simulink model "Smart_Servo_Test"  (R2022b)
settings: Solver=FixedStepAuto  StartTime=0.0  StopTime=10  FixedStep=1e-3  RelTol=1e-3  EnableMultiTasking=on
undefined symbols (not defined in the file or in its folder): AS5600, INA219
libraries: arduinolib x16, simulink x5, hdlsllib x2, dspsigops x2, simulink_extras x1, spsTriangleGeneratorLib x1
settings Model: ExtModeTrigDuration=2  Creator=gotta  LastModifiedBy=gotta
settings SolverCC: AutoInsertRateTranBlk=on
settings DataIOCC: SaveFormat=Array  SaveOutput=off  DSMLogging=off  SaveTime=off  ReturnWorkspaceOutputs=off
settings OptimizationCC: EnhancedBackFolding=on  PassReuseOutputArgsAs=Individual arguments  ZeroExternalMemoryAtStartup=off  ZeroInternalMemoryAtStartup=off  MaxStackSize=64  OptimizeBlockOrder=speed  DifferentSizesBufferReuse=on  OptimizationCustomize=off  EfficientTunableParamExpr=on
settings DebuggingCC: ParameterTunabilityLossMsg=error
settings HardwareCC: ProdBitPerPointer=32  ProdBitPerSizeT=32  ProdBitPerPtrDiffT=32  ProdLargestAtomicInteger=Long  ProdLargestAtomicFloat=Double  ProdWordSize=32  ProdHWDeviceType=ARM Compatible->ARM Cortex
settings SFSimCC: MATLABDynamicMemAlloc=off
settings RTWCC: Description=Embedded Coder  SystemTargetFile=ert.tlc  HardwareBoard=ESP32-WROOM(Arduino Compatible)  TLCOptions="-aInlineSetEventsForThisBaseRateFcn=TLC_FALSE -aSuppressMultiTaskScheduler=TLC_FALSE  -aRateBasedStepFcn=0"  TemplateMakefile=ert_default_tmf  Toolchain=ESP32  BuildConfiguration=Faster Runs
settings CodeAppCC: ForceParamTrailComments=on  IgnoreCustomStorageClasses=off  OperatorAnnotations=on  SimulinkDataObjDesc=on  SFDataObjDesc=on  InsertBlockDesc=on
settings ERTTargetCC: TargetLangStandard=C99 (ISO)  SupportContinuousTime=on  SupportVariableSizeSignals=on  ExtModeTransport=3  ExtModeStaticAlloc=on  ExtModeAutomaticAllocSize=off  ExtModeStaticAllocSize=65536  ExtModeMexFile=ext_xcp  ExtModeIntrfLevel=Level2 - Open

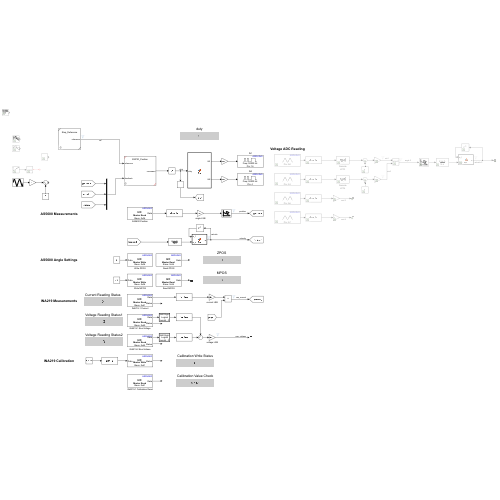
[thumbnail: Simulink's stored preview of the top-level diagram]
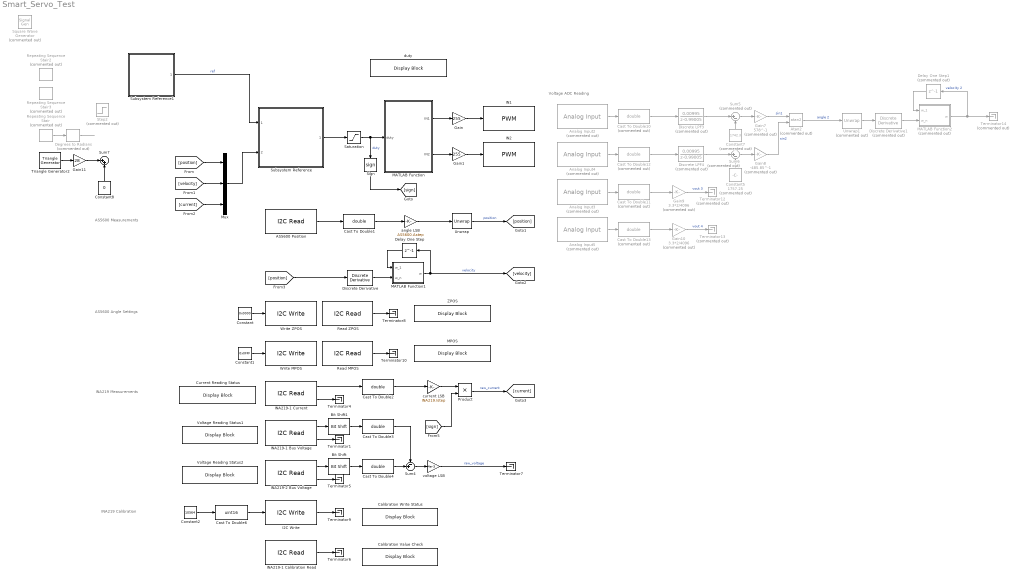
== system Smart_Servo_Test ==
  note: INA219 Calibration
  note: INA219 Measurements
  note: AS5600 Measurements
  note: Voltage ADC Reading
  note: AS5600 Angle Settings
  AS5600 Position : arduinolib/I2C Read  I2CModule=0  Mode=Master  SlaveAddress=AS5600.DEV_ADDR  SlaveByteOrder=BigEndian  Direction=Receiver  RegisterAddressMode=on  RegisterAddress=AS5600.ANGLE_ADDR  SlaveDataType=int16  DataLength=1  NoAck=off  RepeatedStart=off  OutputStatus=off  blockPlatform=ARDUINO  SampleTime=1e-3
  Analog Input2 : arduinolib/Analog Input  Commented=on  pinNumber=0  ReadResultsOnly=off  ConversionTriggerSource=Software  ExternalTriggerType=uint32( 0 )  OutputDataType=uint16  EnableConversionCompleteNotify=off  EnableOuputStatus=off  SampleTime=1e-3  blockPlatform=arduino
  Analog Input3 : arduinolib/Analog Input  Commented=on  pinNumber=6  ReadResultsOnly=off  ConversionTriggerSource=Software  ExternalTriggerType=uint32( 0 )  OutputDataType=uint16  EnableConversionCompleteNotify=off  EnableOuputStatus=off  SampleTime=1e-3  blockPlatform=arduino
  Analog Input4 : arduinolib/Analog Input  Commented=on  pinNumber=3  ReadResultsOnly=off  ConversionTriggerSource=Software  ExternalTriggerType=uint32( 0 )  OutputDataType=uint16  EnableConversionCompleteNotify=off  EnableOuputStatus=off  SampleTime=1e-3  blockPlatform=arduino
  Analog Input5 : arduinolib/Analog Input  Commented=on  pinNumber=7  ReadResultsOnly=off  ConversionTriggerSource=Software  ExternalTriggerType=uint32( 0 )  OutputDataType=uint16  EnableConversionCompleteNotify=off  EnableOuputStatus=off  SampleTime=1e-3  blockPlatform=arduino
  Atan2 : Trigonometry  Commented=on  Operator=atan2
  Bit Shift : hdlsllib/Logic and Bit Operations/Bit Shift  mode=Shift Right Logical  N=3
  Bit Shift1 : hdlsllib/Logic and Bit Operations/Bit Shift  mode=Shift Right Logical  N=3
  Calibration Value Check : DisplayBlock  LabelPosition=Hide  Transparency=1
  Calibration Write Status : DisplayBlock  LabelPosition=Hide  Transparency=1
  Cast To Double{1..4} (4 alike) : DataTypeConversion  OutDataTypeStr=double  SaturateOnIntegerOverflow=off  RndMeth=Floor
  Cast To Double{10..13} (4 alike) : DataTypeConversion  Commented=on  OutDataTypeStr=double  SaturateOnIntegerOverflow=off  RndMeth=Floor
  Cast To Double6 : DataTypeConversion  OutDataTypeStr=uint16  SaturateOnIntegerOverflow=off  RndMeth=Floor
  Constant : Constant  Value=0x0000
  Constant1 : Constant  Value=0x0FFF
  Constant2 : Constant  Value=10564  SampleTime=1e-3
  Constant5 : Constant  Commented=on  Value=1757.25
  Constant7 : Constant  Commented=on  Value=1742.3
  Constant8 : Constant  Value=0
  Current Reading Status : DisplayBlock  LabelPosition=Hide  Transparency=1
  Degrees to Radians : simulink_extras/Transformations/Degrees to Radians  Commented=on
  Delay One Step : Delay  DelayLength=1
  Delay One Step1 : Delay  Commented=on  DelayLength=1
  Discrete LPF3 : DiscreteTransferFcn  Commented=on  Numerator=[0.00995]  Denominator=[1 -0.99005]  SampleTime=1e-3
  Discrete LPF4 : DiscreteTransferFcn  Commented=on  Numerator=[0.00995]  Denominator=[1 -0.99005]  SampleTime=1e-3
  Discrete Derivative : simulink/Discrete/Discrete Derivative  gainval=1.0  ICPrevScaledInput=0.0  OutMin=[]  OutMax=[]  OutDataType=fixdt(1, 16)  OutScaling=2^-10  DoSatur=off
  Discrete Derivative1 : simulink/Discrete/Discrete Derivative  Commented=on  gainval=1.0  ICPrevScaledInput=0.0  OutMin=[]  OutMax=[]  OutDataType=fixdt(1, 16)  OutScaling=2^-10  DoSatur=off
  Gain : Gain  Gain=255
  Gain1 : Gain  Gain=255
  Gain10 : Gain  Commented=on  Gain=3.3*2/4096
  Gain11 : Gain  Gain=28
  Gain7 : Gain  Commented=on  Gain=578^-1
  Gain8 : Gain  Commented=on  Gain=-485.85^-1
  Gain9 : Gain  Commented=on  Gain=3.3*2/4096
  I2C Write : arduinolib/I2C Write  I2CModule=0  Mode=Master  SlaveAddress=0x41  SlaveByteOrder=BigEndian  Direction=Transmitter  RegisterAddressMode=on  RegisterAddress=INA219.CAL_ADDR  SlaveDataType=uint8  DataLength=1  NoAck=off  RepeatedStart=off  OutputStatus=on  blockPlatform=ARDUINO
  IN1 : arduinolib/PWM  pinNumber=16  frequencyType=Specify  desiredFrequency=5e4  achievableFrequency=50000
  IN2 : arduinolib/PWM  pinNumber=4  frequencyType=Specify  desiredFrequency=5e4  achievableFrequency=50000
  INA219-1 Bus Voltage : arduinolib/I2C Read  I2CModule=0  Mode=Master  SlaveAddress=0x40  SlaveByteOrder=BigEndian  Direction=Receiver  RegisterAddressMode=on  RegisterAddress=INA219.BV_ADDR  SlaveDataType=uint16  DataLength=1  NoAck=off  RepeatedStart=off  OutputStatus=on  blockPlatform=ARDUINO  SampleTime=1e-3
  INA219-1 Calibration Read : arduinolib/I2C Read  I2CModule=0  Mode=Master  SlaveAddress=0x41  SlaveByteOrder=BigEndian  Direction=Receiver  RegisterAddressMode=on  RegisterAddress=INA219.CAL_ADDR  SlaveDataType=int16  DataLength=1  NoAck=off  RepeatedStart=off  OutputStatus=off  blockPlatform=ARDUINO  SampleTime=1e-3
  INA219-1 Current : arduinolib/I2C Read  I2CModule=0  Mode=Master  SlaveAddress=0x41  SlaveByteOrder=BigEndian  Direction=Receiver  RegisterAddressMode=on  RegisterAddress=INA219.I_ADDR  SlaveDataType=int16  DataLength=1  NoAck=off  RepeatedStart=off  OutputStatus=on  blockPlatform=ARDUINO  SampleTime=1e-3
  INA219-2 Bus Voltage : arduinolib/I2C Read  I2CModule=0  Mode=Master  SlaveAddress=0x45  SlaveByteOrder=BigEndian  Direction=Receiver  RegisterAddressMode=on  RegisterAddress=INA219.BV_ADDR  SlaveDataType=uint16  DataLength=1  NoAck=off  RepeatedStart=off  OutputStatus=on  blockPlatform=ARDUINO  SampleTime=1e-3
  MATLAB Function : MATLAB Function  TreatAsAtomicUnit=on
  MATLAB Function1 : MATLAB Function  TreatAsAtomicUnit=on
  MATLAB Function2 : MATLAB Function  Commented=on  TreatAsAtomicUnit=on
  MPOS : DisplayBlock  LabelPosition=Hide  Transparency=1
  Mux : Mux  Inputs=3
  Product : Product
  Read MPOS : arduinolib/I2C Read  I2CModule=0  Mode=Master  SlaveAddress=AS5600.DEV_ADDR  SlaveByteOrder=BigEndian  Direction=Receiver  RegisterAddressMode=on  RegisterAddress=0X03  SlaveDataType=uint16  DataLength=1  NoAck=off  RepeatedStart=off  OutputStatus=off  blockPlatform=ARDUINO  SampleTime=1e-3
  Read ZPOS : arduinolib/I2C Read  I2CModule=0  Mode=Master  SlaveAddress=AS5600.DEV_ADDR  SlaveByteOrder=BigEndian  Direction=Receiver  RegisterAddressMode=on  RegisterAddress=0X01  SlaveDataType=uint16  DataLength=1  NoAck=off  RepeatedStart=off  OutputStatus=off  blockPlatform=ARDUINO  SampleTime=1e-3
  Repeating Sequence Stair : simulink/Sources/Repeating Sequence Stair  Commented=on  OutValues=2:2:360  tsamp=2  OutMin=[]  OutMax=[]  OutDataTypeStr=double  OutputDataTypeScalingMode=double  OutDataType=fixdt(0,8)  ConRadixGroup=Best Precision: Vector-wise  OutScaling=2^-12
  Repeating Sequence Stair2 : simulink/Sources/Repeating Sequence Stair  Commented=on  OutValues=[0.1:0.1:1, -[0.1:0.1:1]]  tsamp=10  OutMin=[]  OutMax=[]  OutDataTypeStr=double  OutputDataTypeScalingMode=double  OutDataType=fixdt(0,8)  ConRadixGroup=Best Precision: Vector-wise  OutScaling=2^-12
  Repeating Sequence Stair3 : simulink/Sources/Repeating Sequence Stair  Commented=on  OutValues=[0, 0.5:0.5:10, -[0.5:0.5:10]]  tsamp=5  OutMin=[]  OutMax=[]  OutDataTypeStr=double  OutputDataTypeScalingMode=double  OutDataType=fixdt(0,8)  ConRadixGroup=Best Precision: Vector-wise  OutScaling=2^-12
  Saturation : Saturate  UpperLimit=1  LowerLimit=-1
  Sign : Signum
  Square Wave Generator : SignalGenerator  Commented=on  WaveForm=square  Amplitude=pi  Frequency=0.5
  Step2 : Step  Commented=on  Time=2  After=pi  SampleTime=0
  Subsystem Reference : Subsystem  ReferencedSubsystem=SWPID_Position  Kp=10  Ki=0.9  Kd=0.1
  Subsystem Reference1 : Subsystem  ReferencedSubsystem=Step_Reference  After=pi*10  Time=2
  Sum4 : Sum  Inputs=-+|
  Sum5 : Sum  Commented=on  Inputs=|+-
  Sum6 : Sum  Commented=on  Inputs=|+-
  Sum7 : Sum  Inputs=|++
  Terminator{1,4..10} (8 alike) : Terminator
  Terminator12 : Terminator  Commented=on
  Terminator13 : Terminator  Commented=on
  Terminator14 : Terminator  Commented=on
  Triangle Generator2 : spsTriangleGeneratorLib/Triangle Generator  Freq=0.05  Phase=90  Ts=0
  Unwrap : dspsigops/Unwrap  tol=pi  InputProcessing=Columns as channels (frame based)  running=off
  Unwrap1 : dspsigops/Unwrap  Commented=on  tol=pi  InputProcessing=Columns as channels (frame based)  running=off
  Voltage Reading Status1 : DisplayBlock  LabelPosition=Hide  Transparency=1
  Voltage Reading Status2 : DisplayBlock  LabelPosition=Hide  Transparency=1
  Write MPOS : arduinolib/I2C Write  I2CModule=0  Mode=Master  SlaveAddress=0x36  SlaveByteOrder=BigEndian  Direction=Transmitter  RegisterAddressMode=on  RegisterAddress=0X03  SlaveDataType=uint8  DataLength=1  NoAck=off  RepeatedStart=off  OutputStatus=off  blockPlatform=ARDUINO
  Write ZPOS : arduinolib/I2C Write  I2CModule=0  Mode=Master  SlaveAddress=0x36  SlaveByteOrder=BigEndian  Direction=Transmitter  RegisterAddressMode=on  RegisterAddress=0X01  SlaveDataType=uint8  DataLength=1  NoAck=off  RepeatedStart=off  OutputStatus=off  blockPlatform=ARDUINO
  ZPOS : DisplayBlock  LabelPosition=Hide  Transparency=1
  angle LSB : Gain  Gain=AS5600.Astep
  current LSB : Gain  Gain=INA219.Istep
  duty : DisplayBlock  LabelPosition=Hide  Transparency=1
  voltage LSB : Gain  Gain=4e-3
  wires:
  Cast To Double2/1 -> current LSB/1
  INA219-1 Current/1 -> Cast To Double2/1
  Cast To Double1/1 -> angle LSB/1
  angle LSB/1 -> Unwrap/1
  INA219-1 Current/2 -> Terminator4/1
  INA219-1 Calibration Read/1 -> Terminator6/1
  Cast To Double6/1 -> I2C Write/1
  I2C Write/1 -> Terminator9/1
  [position] -> Mux/1
  [current] -> Mux/3
  MATLAB Function1/1(w) -> [velocity], Delay One Step/1  "velocity"
  AS5600 Position/1 -> Cast To Double1/1
  Mux/1 -> Subsystem Reference/2
  Gain1/1 -> IN2/1
  Gain/1 -> IN1/1
  MATLAB Function/1(IN1) -> Gain/1
  MATLAB Function/2(IN2) -> Gain1/1
  Saturation/1 -> Sign/1, MATLAB Function/1(duty)  "duty"
  Constant2/1 -> Cast To Double6/1
  Analog Input2/1 -> Cast To Double10/1
  Analog Input3/1 -> Cast To Double11/1
  Analog Input5/1 -> Cast To Double13/1
  Analog Input4/1 -> Cast To Double12/1
  Cast To Double11/1 -> Gain9/1
  Cast To Double13/1 -> Gain10/1
  Sign/1 -> [sign]
  Read ZPOS/1 -> Terminator8/1
  Read MPOS/1 -> Terminator10/1
  Constant/1 -> Write ZPOS/1
  Constant1/1 -> Write MPOS/1
  Gain9/1 -> Terminator12/1  "vout 3"
  Gain10/1 -> Terminator13/1  "vout 4"
  INA219-1 Bus Voltage/2 -> Terminator1/1
  INA219-2 Bus Voltage/2 -> Terminator5/1
  INA219-2 Bus Voltage/1 -> Bit Shift/1
  INA219-1 Bus Voltage/1 -> Bit Shift1/1
  Cast To Double3/1 -> Sum4/1
  Cast To Double4/1 -> Sum4/2
  Degrees to Radians/1 -> ?
  [position] -> Discrete Derivative/1
  Cast To Double10/1 -> Discrete LPF3/1
  Cast To Double12/1 -> Discrete LPF4/1
  Discrete LPF3/1 -> Sum5/1
  Discrete LPF4/1 -> Sum6/1
  Sum5/1 -> Gain7/1
  Sum6/1 -> Gain8/1
  Constant5/1 -> Sum6/2
  Constant7/1 -> Sum5/2
  Gain7/1 -> Atan2/1  "sin1"
  Gain8/1 -> Atan2/2  "sin2"
  Atan2/1 -> Unwrap1/1  "angle 2"
  Unwrap1/1 -> Discrete Derivative1/1
  Discrete Derivative/1 -> MATLAB Function1/2(w_n)
  Delay One Step/1 -> MATLAB Function1/1(w_1)
  Discrete Derivative1/1 -> MATLAB Function2/2(w_n)
  MATLAB Function2/1(w) -> Delay One Step1/1, Terminator14/1  "velocity 2"
  Delay One Step1/1 -> MATLAB Function2/1(w_1)
  Product/1 -> [current]  "raw_current"
  Sum4/1 -> voltage LSB/1
  voltage LSB/1 -> Terminator7/1  "raw_voltage"
  Triangle Generator2/1 -> Gain11/1
  Gain11/1 -> Sum7/1
  Constant8/1 -> Sum7/2
  Bit Shift/1 -> Cast To Double4/1
  Bit Shift1/1 -> Cast To Double3/1
  Repeating Sequence Stair/1 -> Degrees to Radians/1
  [sign] -> Product/2
  current LSB/1 -> Product/1
  Unwrap/1 -> [position]  "position"
  [velocity] -> Mux/2
  Subsystem Reference1/1 -> Subsystem Reference/1  "ref"
  Subsystem Reference/1 -> Saturation/1

== matlab function Smart_Servo_Test/MATLAB Function ==
  data: duty input; IN1 output; IN2 output
function [IN1, IN2] = fcn(duty)
% go from movement to brake, not from movement to coast

if duty > 0
    % forward movement
    IN1 = 1 - abs(duty);
    IN2 = 1;
elseif duty < 0
    % reverse movement
    IN1 = 1;
    IN2 = 1 - abs(duty);
else
    % any other case -> brake
    IN1 = 1;
    IN2 = 1;
end

% temp = IN1;
% IN1 = 1 - IN2;
% IN2 = 1 - temp;

== matlab function Smart_Servo_Test/MATLAB Function2 ==
  data: w_1 input; w output; w_n input
function w = fcn(w_1, w_n)

if abs(w_n-w_1) > 100
    w = w_1;
else
    w = w_n;
end

== matlab function Smart_Servo_Test/MATLAB Function1 ==
  data: w_1 input; w output; w_n input
function w = fcn(w_1, w_n)

if abs(w_n-w_1) > 100
    w = w_1;
else
    w = w_n;
end
